simulink model "TRUAV_Dynamics_from_GTRS_trim"  (R2022b)
settings: Solver=ode4  StartTime=0.0  StopTime=3  FixedStep=0.004  RelTol=1e-3
values from neighbouring files (symbols this model uses):
  a_sound = 1116.45    [init_0_GTRS_data_Run_this_file.m]
  alpha_F_rad = alpha_F_deg * (pi/180)    [init_Vetical_2_Table.m]
  alpha_F_rad_table = alpha_F_table * (pi/180)    [init_Fuselage_Aero_Table.m]
  alpha_H_rad = alpha_H_deg * (pi/180)    [init_Horizontal_Table.m]
  alpha_HD_rad = alpha_HD_deg * (pi/180)    [init_Horizontal_C_D_Table.m]
  alpha_r0 = 0    [init_0_GTRS_data_Run_this_file.m]
  alpha_WF_epsilon_M_rad = alpha_WF_deg * pi/180    [init_WingWake_Deflection_Table.m]
  alpha_WS_CL_rad = alpha_WS_CL_deg * (pi/180)    [init_Wing_Slide_Table.m]
  b_w = 32.17    [init_0_GTRS_data_Run_this_file.m]
  beta_F_rad = beta_F_deg * (pi/180)    [init_Vetical_2_Table.m]
  beta_LD_rad_table = beta_LD_table * (pi/180)    [init_Fuselage_Aero_Table.m]
  beta_m_epsilon_M_rad = beta_m_deg * pi/180    [init_WingWake_Deflection_Table.m]
  beta_m_rad_cn = beta_m_deg_cn * pi/180    [init_Wing_Free_Table.m]
  beta_M_rad_table = beta_M_table  * (pi/180)    [init_Fuselage_Aero_Table.m]
  beta_m_S_rad = beta_m_S_deg * (pi/180)    [init_Vetical_2_Table.m]
  beta_m_WS_CL_rad = beta_m_WS_CL_deg * (pi/180)    [init_Wing_Slide_Table.m]
  beta_rad_brk = beta_KBR_rad    [init_Vetical_2_Table.m]
  beta_v_rad = beta_v_deg * (pi/180)    [init_Vetical_1_Table.m]
  beta_vD_rad = beta_vD_deg * (pi/180)    [init_Vetical_1_Table.m]
  beta_WF_Cl_rad = beta_W_deg * (pi/180)    [init_Wing_Free_Table.m]
  beta_WF_CL_rad = beta_CL_deg * (pi/180)    [init_Wing_Free_Table.m]
  beta_YlN_rad_table = beta_YlN_table * (pi/180)    [init_Fuselage_Aero_Table.m]
  c_HW = 3.92    [init_0_GTRS_data_Run_this_file.m]
  C_l_beta_CLwp_table = [ ... (first row only)    [init_Wing_Free_Table.m]
  C_l_beta_pro_CLwp_table = [ ... (first row only)    [init_Wing_Free_Table.m]
  C_L_delta_a_table = [0.00316, 0.00396, 0.00476, 0]    [init_Wing_Free_Table.m]
  C_LHB = -0.00422    [init_0_GTRS_data_Run_this_file.m]
  C_lp_C_LWP = -0.774    [init_0_GTRS_data_Run_this_file.m]
  C_m_wp_table = [ ... (first row only)    [init_Wing_Free_Table.m]
  C_MHA = 0    [init_0_GTRS_data_Run_this_file.m]
  C_MHO = 0    [init_0_GTRS_data_Run_this_file.m]
  c_R = 14/12    (= 1.16666666667)    [init_0_GTRS_data_Run_this_file.m]
  c_w = 5.225    [init_0_GTRS_data_Run_this_file.m]
  C_Y_beta = 0    [init_0_GTRS_data_Run_this_file.m]
  CD0_high_Mach_data = [0.0177, 0.0178, 0.0179, 0.0405]    [init_Wing_Free_Table.m]
  CD_4D_table = zeros(49, 4, 2, 4)    [init_Wing_Slide_Table.m]
  CDH_2D_table = zeros(length(alpha_HD_deg), length(mach_vec))    [init_Horizontal_C_D_Table.m]
  CDV_2D_table = zeros(length(beta_vD_deg), length(mach_vec))    [init_Vetical_1_Table.m]
  CL_4D_table = zeros(49, 4, 2, 4)    [init_Wing_Slide_Table.m]
  CLH_3D_table = zeros(length(alpha_H_deg), length(delta_e_deg), length(mach_vec))    [init_Horizontal_Table.m]
  CYV_3D_table = zeros(length(beta_v_deg), length(delta_r_deg), length(mach_vec))    [init_Vetical_1_Table.m]
  D_alpha_table = [D_part1, D_part2, D_part3, D_part4]    [init_Fuselage_Aero_Table.m]
  D_beta_table = [ fliplr(D_beta_half(2:end)),  D_beta_half]    [init_Fuselage_Aero_Table.m]
  D_ke = 0.24    [init_0_GTRS_data_Run_this_file.m]
  D_Kr = 0.24    [init_0_GTRS_data_Run_this_file.m]    (also in init_Vetical_1_Table.m)
  DBFO = -1.56    [init_0_GTRS_data_Run_this_file.m]
  delta_e_rad = delta_e_deg * (pi/180)    [init_Horizontal_Table.m]
  delta_r_deg = [-20, -15, 0, 15, 20]    [init_Vetical_1_Table.m]
  DLANG = -0.5    [init_0_GTRS_data_Run_this_file.m]
  epsilon_W_table = permute(epsilon_W_3D, [3, 1, 2])    [init_WingWake_Deflection_Table.m]
  flap_rad = flap_deg * (pi/180)    [init_Wing_Free_Table.m]    (also in init_Wing_Slide_Table.m)
  ft2m = 0.3048    [init_0_GTRS_data_Run_this_file.m]
  h_HW = [-0.5838, 0.01158, 0.5967, 0.002547,-2.2519]    [init_0_GTRS_data_Run_this_file.m]
  I_b = 102.5    [init_0_GTRS_data_Run_this_file.m]
  i_H = 0    [init_0_GTRS_data_Run_this_file.m]
  i_v = 0    [init_0_GTRS_data_Run_this_file.m]
  i_w = 0    [init_0_GTRS_data_Run_this_file.m]
  in2ft = 1/12    (= 0.0833333333333)    [init_0_GTRS_data_Run_this_file.m]
  Ixx = 52795    [init_0_GTRS_data_Run_this_file.m]
  Ixz = 1234    [init_0_GTRS_data_Run_this_file.m]
  Iyy = 21360    [init_0_GTRS_data_Run_this_file.m]
  Izz = 66335    [init_0_GTRS_data_Run_this_file.m]
  K1delta_data = [ ... (first row only)    [init_Wing_Free_Table.m]
  K_coeffs = [1.6 0]    [init_0_GTRS_data_Run_this_file.m]
  K_FWDF = -0.0035    [init_0_GTRS_data_Run_this_file.m]
  K_FWO = 1.4    [init_0_GTRS_data_Run_this_file.m]
  K_HNU = 0.8    [init_0_GTRS_data_Run_this_file.m]
  K_vNU = 1    [init_Vetical_1_Table.m]
  KBR_table = KBR_table_full    [init_Vetical_2_Table.m]
  Kn_delta_data = [ ... (first row only)    [init_Wing_Free_Table.m]
  Kno_delta_data = [ ... (first row only)    [init_Wing_Free_Table.m]
  L_alpha_table = [L_part1, L_part2, L_part3, L_part4]    [init_Fuselage_Aero_Table.m]
  L_beta_table = [ fliplr(L_beta_half(2:end)),  L_beta_half]    [init_Fuselage_Aero_Table.m]
  l_beta_table = [l_beta_neg, l_beta_pos]    [init_Fuselage_Aero_Table.m]
  L_n = 4.667    [init_0_GTRS_data_Run_this_file.m]
  lambda_w = -6.5*deg2rad    (= -0.11344640138)    [init_0_GTRS_data_Run_this_file.m]
  LBFO = -7.23    [init_0_GTRS_data_Run_this_file.m]
  LLANG = 0    [init_0_GTRS_data_Run_this_file.m]
  m2ft = 1/ft2m    (= 3.28083989501)    [init_0_GTRS_data_Run_this_file.m]
  M_alpha_table = [M_part1, M_part2, M_part3, M_part4]    [init_Fuselage_Aero_Table.m]
  M_beta_table = [ fliplr(M_beta_half(2:end)), M_beta_half]    [init_Fuselage_Aero_Table.m]
  Mach_brk = [0.2, 0.4, 0.5, 0.6]    [init_Wing_Free_Table.m]
  mach_vec = [0.2, 0.4, 0.5, 0.6]    [init_Horizontal_C_D_Table.m]    (also in init_Horizontal_Table.m; init_Vetical_1_Table.m)
  mass = 403.7    [init_0_GTRS_data_Run_this_file.m]
  mast_rad = mast_deg * pi/180    [init_Wing_Free_Table.m]
  MBFO = 66.5    [init_0_GTRS_data_Run_this_file.m]
  Mn_X_ke = [0 0.2 0.4 0.5 0.6 0.7]    [init_Horizontal_Table.m]
  N_beta_table = [N_beta_neg, N_beta_pos]    [init_Fuselage_Aero_Table.m]
  pos_x_CG = 300    [init_0_GTRS_data_Run_this_file.m]
  pos_x_H = 300    [init_0_GTRS_data_Run_this_file.m]
  pos_x_HW = 560    [init_0_GTRS_data_Run_this_file.m]
  pos_x_Nac = 291.7    [init_0_GTRS_data_Run_this_file.m]
  pos_x_V = 570    [init_0_GTRS_data_Run_this_file.m]
  pos_x_W = 291.7    [init_0_GTRS_data_Run_this_file.m]
  pos_y_CG = 0    [init_0_GTRS_data_Run_this_file.m]
  pos_y_H = 193    [init_0_GTRS_data_Run_this_file.m]
  pos_y_HW = 0    [init_0_GTRS_data_Run_this_file.m]
  pos_y_Nac = 193    [init_0_GTRS_data_Run_this_file.m]
  pos_y_V = 115.69    [init_0_GTRS_data_Run_this_file.m]
  pos_y_W = 96.6    [init_0_GTRS_data_Run_this_file.m]
  pos_z_CG = 81.65    [init_0_GTRS_data_Run_this_file.m]
  pos_z_H = 100    [init_0_GTRS_data_Run_this_file.m]
  pos_z_HW = 103    [init_0_GTRS_data_Run_this_file.m]
  pos_z_Nac = 118    [init_0_GTRS_data_Run_this_file.m]
  pos_z_V = 77    [init_0_GTRS_data_Run_this_file.m]
  pos_z_W = 96    [init_0_GTRS_data_Run_this_file.m]
  R = 12.5    [init_0_GTRS_data_Run_this_file.m]
  rho = 0.002376    [init_0_GTRS_data_Run_this_file.m]
  s_HW = 50.25    [init_0_GTRS_data_Run_this_file.m]
  S_max = 56    [init_0_GTRS_data_Run_this_file.m]
  S_v = 20.25    [init_0_GTRS_data_Run_this_file.m]
  S_w = 181    [init_0_GTRS_data_Run_this_file.m]
  Sidewash_4D = zeros(length(alpha_F_deg), length(beta_F_deg), length(beta_m_S_deg), length(delta_F_S_deg))    [init_Vetical_2_Table.m]
  slugft2kgm = 1.35582    [init_0_GTRS_data_Run_this_file.m]
  tau_e = 0.518    [init_0_GTRS_data_Run_this_file.m]
  tau_r = 0.27    [init_0_GTRS_data_Run_this_file.m]    (also in init_Vetical_1_Table.m)
  theta_0_R = 0.750    (= 0.75)    [init_0_GTRS_data_Run_this_file.m]
  theta_0_W = 1.187    [init_0_GTRS_data_Run_this_file.m]
  theta_twist = -41*deg2rad    (= -0.715584993318)    [init_0_GTRS_data_Run_this_file.m]
  u_max = 1181/12    (= 98.4166666667)    [init_0_GTRS_data_Run_this_file.m]
  ... (+3 more)
undefined symbols (not defined in the file or in its folder): beta_m_rad, F, Light, MIL, sigbuilder_block, tilt_cmd
libraries: simulink x2, sharedtransform x2, aerolibasang x2, aerolibwind2 x1
(part 3 of 4)

== matlab function TRUAV_Dynamics_from_GTRS_trim/Force and Moments/Propulsion1/Rotor Assembly 2 left/叶素法 ==
  data: para input; V_H input; r_n input; beta_F_params input; Psi_1 input; v_i input; a_MR input; F_b output; M_b output; delta_H input; T_NAC2B input; T_H2NAC input; ABC input; Thrust_mag output
function [F_b, M_b, Thrust_mag] = forces_moments_Left(para, V_H, r_n, beta_F_params, Psi_1, ...
                                          v_i, a_MR, delta_H, T_NAC2B, T_H2NAC,ABC)
    % ========== 左旋翼（CW）全叶素积分气动力与力矩计算 ==========
    R = para(1); theta_twist = para(2);
    rho = para(3); c = para(4); a_sound = para(5); Nb = 3;                
    
    % 同样内部取反横向周期变距，以匹配飞行控制逻辑
    theta_all = ABC(1);
    A1 = -ABC(2); B1 = ABC(3); 
    
    a0 = beta_F_params(1); a1s = beta_F_params(2); b1s = beta_F_params(3);
    delta_H = delta_H(:); % 强行拉直为 3x1 列向量
    
    N_segments = 40;
    dr = R / N_segments;
    r_vec = (0.5:1:N_segments-0.5)' * dr; 
    x = r_vec / R;
    
   % 初始化整个旋翼在桨毂系(Hub)下的总力和总力矩
    F_HUB_total = zeros(3,1); 
    M_HUB_total = zeros(3,1); 
    
    % ========== 改造点：方位角离散平均法 ==========
    N_azimuth = 36; % 将一圈分为 36 份 (每 10 度算一次)
    dPsi = 2 * pi / N_azimuth;
    
    for k = 1:N_azimuth
        % 虚拟桨叶当前的方位角
        Psi = (k - 1) * dPsi; 
        
        % 根据傅里叶级数实时计算该方位角下的挥舞角和角速度
        beta = a0 - a1s*cos(Psi) - b1s*sin(Psi);
        beta_dot = r_n * (a1s*sin(Psi) - b1s*cos(Psi));
        
        dY_prime = zeros(N_segments, 1);
        dZ_prime = zeros(N_segments, 1);
        dQ_torque = zeros(N_segments, 1); 
        
        % ========== 2. 逐段计算叶素气动力 ==========
        for i = 1:N_segments
            r_local = r_vec(i);
            
            % 【左旋翼 CW 的正确面内速度分解】
            % 注意这里和右旋翼的区别！
            U_T = r_n * r_local + V_H(1) * sin(Psi) - V_H(2) * cos(Psi); 
            U_R = V_H(1) * cos(Psi) + V_H(2) * sin(Psi);
            
            U_P = r_local * beta_dot + U_R * beta + V_H(3) + v_i;
            
            if U_T < 0; U_T = abs(U_T); end
            
            phi_b = atan2(U_P, U_T);
            % 注意：左旋翼在函数开头应该已经把 A1 内部取反了 (A1 = -ABC(2))
            theta = theta_all + A1*cos(Psi) + B1*sin(Psi) + theta_twist*x(i);
            alpha_blade = theta - phi_b;
            
            U = sqrt(U_T^2 + U_P^2);
            M_local = U / a_sound;
            abs_alpha = abs(alpha_blade);
            
            % 阻力系数经验公式
            cd_base = 0.015 + abs_alpha * (0.068 + abs_alpha * 0.81);
            comp_term = 0.01 * abs_alpha + 0.02 *(0.85+ max(M_local,0.35)); 
            cd_comp = max(0, comp_term);
            cd_local = min(0.11, cd_base + cd_comp);
            
            dL = 0.5 * rho * U^2 * a_MR * alpha_blade * c * dr;
            dD = 0.5 * rho * U^2 * cd_local * c * dr;
            
            % 桨叶主轴系气动力
            dY_prime(i) = dL * sin(phi_b) + dD * cos(phi_b);
            dZ_prime(i) = dL * cos(phi_b) - dD * sin(phi_b);
            dQ_torque(i) = dY_prime(i) * r_local; 
        end
        
        Y_prime = sum(dY_prime);   
        Z_prime = sum(dZ_prime);   
        Q_blade = sum(dQ_torque);  
        
        % 顺时针旋转的局部受力向量 (阻力始终与切向速度相反)
        F_blade_local = [0; -Y_prime; Z_prime]; 
        
        % ========== 3. 坐标转换：桨叶系 -> 挥舞系 -> 桨毂系 ==========
        
        % 3.1 【已修复】挥舞矩阵 (绕 Y 轴向上翘起 beta)
        T_Flap2Rot = [ cos(beta),  0, -sin(beta);
                               0,  1,          0;
                       sin(beta),  0,  cos(beta)];
        
        % 3.2 顺时针(CW)旋转的特征坐标转换矩阵
        T_Rot2Hub = [ cos(Psi), sin(Psi), 0;
                     -sin(Psi), cos(Psi), 0;
                             0,        0, 1];
                        
        % 单根桨叶力转换到桨毂固定系
        F_HUB_blade = T_Rot2Hub * T_Flap2Rot * F_blade_local;
        
        % 累加这个方位角切片上的力
        F_HUB_total = F_HUB_total + F_HUB_blade;

        Thrust_mag = abs(F_HUB_total(3));
        
        % 累加反扭矩：左旋翼(CW)的气动反扭矩阻碍旋转，方向为 +Z
        M_HUB_total(3) = M_HUB_total(3) - Q_blade; 
    end
    
    % ========== 4. 求一圈的平均力，再乘以真实桨叶数 ==========
    % 因为我们积了 36 次，相当于有 36 片桨叶，所以要除以 36，再乘以真实的 3 片
    F_HUB_total = F_HUB_total * (Nb / N_azimuth);
    M_HUB_total = M_HUB_total * (Nb / N_azimuth);
    
    % ========== 5. 转换到机体轴系 (Body Frame) ==========
    T_HUB2BODY = T_NAC2B * T_H2NAC; 
    F_b = T_HUB2BODY * F_HUB_total;
    M_hub_body = T_HUB2BODY * M_HUB_total;
    
    % ========== 6. 计算最终重心的总力矩 ==========
    M_b = M_hub_body + cross(delta_H, F_b);
  end

== matlab function TRUAV_Dynamics_from_GTRS_trim/6DOF Model/disturbance2/noise Disturb1 ==
  data: n input; t input; y output
function y = fcn(n, t)
    if t>=7&&t<=14
        y=n;
    else
        y=0*n;
    end
end

== matlab function TRUAV_Dynamics_from_GTRS_trim/6DOF Model/disturbance2/noise Disturb2 ==
  data: n input; t input; y output
function y = fcn(n, t)
    if t>=19&&t<=23
        y=n;
    else
        y=0*n;
    end
end

== matlab function TRUAV_Dynamics_from_GTRS_trim/Force and Moments/Propulsion1/Rotor Assembly 2 left/旋转矩阵计算 ==
  data: T_H2NAC output; tilt input; T_NAC2B output
function [T_H2NAC ,T_NAC2B]  = Transf(tilt)

T_H2NAC = [-1     0     0;
          0     1     0;
          0     0     -1];

T_NAC2B = [cos(tilt)  0     -sin(tilt);
           0          1       0;
           sin(tilt)  0     cos(tilt)];

== matlab function TRUAV_Dynamics_from_GTRS_trim/6DOF Model/MATLAB Function ==
  data: Ib input; F input; M input; V_b input; wbe_b input; Eu input; d1 input; x1to3dot output; x4to6dot output; x7to9dot output; d2 input
function [x1to3dot,x4to6dot,x7to9dot] = EuFcn(Ib,F,M,V_b,wbe_b,Eu,d1,d2)

p=wbe_b(1);q=wbe_b(2);r=wbe_b(3);
Ix=Ib(1);Iy=Ib(2);Iz=Ib(3);Ixz=Ib(4);
Ibb=[Ix 0 Ixz;
    0 Iy 0;
    Ixz 0 Iz];
Mx = M(1);My = M(2);Mz = M(3);

x7=Eu(1);
x8=Eu(2);
%-----------------10. STATE DERIVATIVES--------------------------    
 %Form F_b (all the forces in Fb) and calculate udot, vdot, wdot
 x1to3dot=(1/403.7)*F-cross(wbe_b,V_b)+(1/403.7)*d1;
 
 %Form Mcg_b (all moment about CoG in Fb) and calculate pdot, qdot, rdot.
%  invIb=inv(Ib);
 x4to6dot=Ibb\(M-cross(wbe_b,Ibb*wbe_b)+d2);
 
 %Calculate phidot, thetadot, and psidot
 R_omega=[1 sin(x7)*tan(x8) cos(x7)*tan(x8);
        0 cos(x7) -sin(x7);
        0 sin(x7)/cos(x8) cos(x7) /cos(x8)];
%  H_phi=[0 cos(x7) -sin(x7);
%         0 sin(x7)/cos(x8) cos(x7) /cos(x8);
%         1 sin(x7)*tan(x8) cos(x7)*tan(x8)];  
 x7to9dot=R_omega*wbe_b;

== matlab function TRUAV_Dynamics_from_GTRS_trim/6DOF Model/MATLAB Function3 ==
  data: R_be output; Par_b input; Par_e output; Eu input
function [R_be,Par_e]= EuFcn(Par_b,Eu)

phi=Eu(1);theta=Eu(2);psi=Eu(3);



R_be = [cos(theta)*cos(psi), sin(phi)*sin(theta)*cos(psi)-cos(phi)*sin(psi), sin(phi)*sin(psi)+cos(phi)*sin(theta)*cos(psi);
        cos(theta)*sin(psi), sin(phi)*sin(theta)*sin(psi)+cos(phi)*cos(psi), -sin(phi)*cos(psi)+cos(phi)*sin(theta)*sin(psi);
        -sin(theta), sin(phi)*cos(theta), cos(phi)*cos(theta)];

Par_e=R_be*Par_b;
 
for i=1:1:9
      if isnan(R_be(i))
         Par_e(i)= double(isnan(Par_e(i)));
      end
end

== matlab function TRUAV_Dynamics_from_GTRS_trim/6DOF Model/disturbance1/Disturb4 ==
  data: t input; y output
function y = fcn(t)
    y=1+2*sin(1.5*pi*t)+cos(0.5*pi*t);
    
end

== matlab function TRUAV_Dynamics_from_GTRS_trim/6DOF Model/disturbance1/Disturb1 ==
  data: t input; y output
function y = fcn(t)
    y=2+1.5*cos(2*pi*t)+sin(0.3*pi*t);
%     if t>=8&&t<=14
%         y=y1*(1+sin(1/6*pi*(t-8)));
%     elseif t>=21&&t<=23
%         y=y1*(1+sin(1/2*pi*(t-21)));
%     else 
%         y=y1;
%     end
end

== matlab function TRUAV_Dynamics_from_GTRS_trim/6DOF Model/disturbance1/Disturb2 ==
  data: t input; y output
function y = fcn(t)
    y=-2+1.5*sin(pi*t)+2*cos(3*pi*t);
%     if t>=8&&t<=14
%         y=y1*(1+sin(1/6*pi*(t-8)));
%     elseif t>=21&&t<=23
%         y=y1*(1+sin(1/2*pi*(t-21)));
%     else 
%         y=y1;
%     end
end

== matlab function TRUAV_Dynamics_from_GTRS_trim/6DOF Model/disturbance1/noise Disturb1 ==
  data: n input; t input; y output
function y = fcn(n, t)
    if t>=7&&t<=14
        y=n;
    else
        y=0*n;
    end
end

== matlab function TRUAV_Dynamics_from_GTRS_trim/6DOF Model/disturbance1/noise Disturb2 ==
  data: n input; t input; y output
function y = fcn(n, t)
    if t>=19&&t<=23
        y=n;
    else
        y=0*n;
    end
end

== matlab function TRUAV_Dynamics_from_GTRS_trim/6DOF Model/限制在±180度 ==
  data: x input; y output
function y = fcn(x)
x = mod(x,2*pi);
y = x.*(0<=x & x <= pi) + (x - 2*pi).*(pi<x & x<2*2*pi);  % x in (-pi,pi]

== matlab function TRUAV_Dynamics_from_GTRS_trim/Force and Moments/body/Fuselage/机身气动力 ==
  data: q_F output; para input; V_body input; alpha_rad output; beta_rad output
function [q_F, alpha_rad, beta_rad] = f_kinematics(para, V_body)
    % =====================================================================
    % 机身拆分模块 1：运动学解算 (算出迎角、侧滑角与动压)
    % ---------------------------------------------------------------------
    % 【输出说明】
    % alpha_rad : 机身迎角 (rad)，输出给外部 Alpha 查表模块
    % beta_rad  : 机身侧滑角 (rad)，输出给外部 Beta 查表模块
    % q_F       : 机身动压 (lb/ft^2)，直接传递给第二个模块
    % =====================================================================
    
    rho = para(1);  
         
    % 计算局部相对速度
    V_local = V_body;
    u = V_local(1); 
    v = V_local(2); 
    w = V_local(3);
    
    V_mag = norm(V_local); 
    
    % 求解角度与动压
    if V_mag < 0.1
        alpha_rad = 0;
        beta_rad  = 0;
        q_F       = 0;
    else
        alpha_rad = atan2(w, u);
        v_ratio = max(min(v / V_mag, 1), -1); 
        beta_rad  = asin(v_ratio);
        q_F = 0.5 * rho * V_mag^2;
    end
end

== matlab function TRUAV_Dynamics_from_GTRS_trim/Force and Moments/body/Fuselage/机身气动力1 ==
  data: para input; q_F input; F_b output; M_b output; alpha_rad input; beta_rad input; aero_alpha input; aero_beta input
function [F_b, M_b] = F_M_f(para, q_F, alpha_rad, beta_rad, aero_alpha, aero_beta)
    % =====================================================================
    % 机身拆分模块 2：动力学合成 (接收查表结果，算出总力和力矩)
    % ---------------------------------------------------------------------
    % 
    % aero_alpha : [3x1] 外部 Alpha 查表结果打包 [L_alpha_0; D_alpha_0; M_alpha_0]
    % aero_beta  : [3x1] 外部 Beta 查表结果打包 [L_beta; D_beta; M_beta]
    % =====================================================================
    
    LBFO  = para(2); 
    LLANG = para(3); 
    DBFO  = para(4); 
    DLANG = para(5); 
    MBFO  = para(6); 
    
    
    
    % 1. 解析外部查表传入的数据
    L_alpha_0 = aero_alpha(1); 
    D_alpha_0 = aero_alpha(2); 
    M_alpha_0 = aero_alpha(3); 
    
    L_beta = aero_beta(1); 
    D_beta = aero_beta(2); 
    M_beta = aero_beta(3); 
    Y_beta = aero_beta(4); 
    l_beta = aero_beta(5); 
    N_beta = aero_beta(6); 
         
    % 2. 核心经验公式计算
    cos2_beta = (cos(beta_rad))^2;
    
    L_F       = q_F * ( L_alpha_0 * cos2_beta + L_beta + LBFO + LLANG );
    D_F       = q_F * ( D_alpha_0 * cos2_beta + D_beta + DBFO + DLANG );
    Y_F_prime = q_F * Y_beta;
    
    M_F_prime = q_F * ( M_alpha_0 * cos2_beta + M_beta + MBFO );
    l_F_prime = q_F * l_beta;
    N_F_prime = q_F * N_beta;
    
    % 3. 风轴向机体轴 3D 转换
    sa = sin(alpha_rad); ca = cos(alpha_rad);
    sb = sin(beta_rad);  cb = cos(beta_rad);
    
    F_body = zeros(3,1);
    F_body(1) = -D_F * ca * cb - Y_F_prime * ca * sb + L_F * sa;
    F_body(2) = -D_F * sb      + Y_F_prime * cb;
    F_body(3) = -D_F * sa * cb - Y_F_prime * sa * sb - L_F * ca;
    
    M_profile = zeros(3,1);
    M_profile(1) =  l_F_prime * ca - N_F_prime * sa;
    M_profile(2) =  M_F_prime; 
    M_profile(3) =  l_F_prime * sa + N_F_prime * ca;
    
    % 4. 平行轴定理向重心搬移
    M_b = M_profile;
    F_b = F_body;
end

== matlab function TRUAV_Dynamics_from_GTRS_trim/Force and Moments/Propulsion1/Rotor Assembly 2 left/计算挥舞角、桨尖马赫数 桨叶升力线斜率1 ==
  data: para input; V input; beta_F_Para output; r_n input; tilt input; mu input; AB input; alpha input; pqr input; v_1d input; M_tip output; a_MR output; lamda input
function [beta_F_Para, M_tip, a_MR] = rotor_cal1(...
    para, V, r_n, tilt, mu, AB, alpha, pqr, v_1d, lamda)
% 整合旋翼气动与挥舞计算模型（包含洛克数自动计算）
% 输入：
%   para     - 参数向量 [R, theta_0_W, theta_0_R, theta_twist, a_sound, alpha_0, rho, c, I_b]
%              R: 旋翼半径 [ft]
%              theta_0_W: 悬停总距 [rad]（对应β_M=0）
%              theta_0_R: 悬停总距 [rad]（对应β_M=90°）
%              theta_twist: 桨叶线性扭转率 [rad]
%              a_sound: 当地声速 [ft/s]
%              alpha_0: 桨叶零升迎角修正 [rad]
%              rho: 空气密度 [slug/ft³]
%              c: 桨叶弦长 [in]（自动转换为ft）
%              I_b: 桨叶挥舞惯性矩 [slug·ft²]
%   V        - 飞机前进速度 [ft/s]
%   r_n      - 展向位置比率（通常为1，代表桨尖）
%   tilt   - 短舱倾角 [rad]
%   mu       - 前进比（无量纲）
%   AB       - 周期变距向量 [A1, B1]  [rad]
%   alpha    - 迎角[rad]
%   gamma_b  - 洛克数（占位符，实际会被覆盖计算，可任意值）
%   pqr      - 机体角速度 [p,q,r] [rad/s]
%   lamda    - 入流比（未使用，保留接口）
%   Psi    - 方位角 [rad]
% 输出：
%   beta_F     - 挥舞角 [rad]
%   M_tip    - 桨尖马赫数
%   a_MR     - 旋翼升力线斜率 [1/rad]

% 解析参数
R = para(1);
theta_0_W = para(2);
theta_0_R = para(3);
theta_twist = para(4);
a_sound = para(5);
alpha_0 = para(6);
rho = para(7);
c = para(8);
I_b = para(9);

p = pqr(1);
q = pqr(2);
A1 = AB(2);
B1 = AB(3);

% ========== 1. 计算桨尖马赫数 M_tip ==========
V_tip = sqrt(V^2 + (r_n*R)^2 + 2*V*r_n*R*cos(tilt));
M_tip = V_tip / a_sound;

% ========== 2. 计算升力线斜率 a_MR（Kleinhesselink 论文）==========
denom = sqrt(1 - (0.75*M_tip)^2 * sin(tilt));
if denom < 1e-6
    denom = 1e-6;
end
 a_MR = (4.95 + mu * (8 + 30*mu)) / denom;

% ========== 3. 计算洛克数 gamma ==========
gamma_b_calc = rho * a_MR * c * R^4 / I_b;   % 无量纲洛克数

% ========== 4. 计算挥舞角 ==========
theta0 = 2*(tilt)/pi * (theta_0_W - theta_0_R) + theta_0_R;
alpha_s = alpha - tilt;

% ... (前面的 M_tip 和 洛克数 计算保持不变) ...

% 4.1 后倒角 a1s（纵向挥舞）- 陀螺耦合项 p, q 符号取反
term1 = (2*mu) / (1 - 0.5*mu^2);
term2 = (4/3)*theta0 + theta_twist + mu*alpha_s - v_1d/(r_n*R);
term3 = - (1 + 1.5*mu^2) / (1 - 0.5*mu^2) * B1;
% 【修正】：q 变正，p 变负
term4 = 16/gamma_b_calc * q / r_n - p / r_n; 
a1s = term1 * term2 + term3 + term4/(1 - 0.5*mu^2);

% 4.2 侧倒角 b1s（横向挥舞）- 陀螺耦合项 p, q 符号取反
term1_b = (2*mu) / (1 + 0.5*mu^2);
term2_b = (4/3) * mu * alpha_0;
term3_b = A1; 
% 【修正】：p 变正，q 变正
term4_b = 16/gamma_b_calc * p / r_n;
term5_b = q / r_n;
b1s = term1_b * term2_b + term3_b + (term4_b + term5_b)/(1 + 0.5*mu^2);

% 锥度角 a0（简化）
gamma_used = gamma_b_calc;   % 使用计算得到的洛克数
a0 = (gamma_used/8) * ((4/3)*theta0*(1 + mu^2) + 2*lamda*mu);

% 挥舞角随方位角变化
beta_F_Para = [a0 a1s b1s];

end

== matlab function TRUAV_Dynamics_from_GTRS_trim/Force and Moments/body/Horizontal/平尾气动力1 ==
  data: para input; CG input; AC_t input; tilt input; Ke_coeffs input; q_H input; alpha_body_t input; F_b output; M_b output; beta_t input; alpha_HL input; C_LH input; C_DH input
function [F_b, M_b] = tail_dynamics(para, CG, AC_t, tilt, Ke_coeffs, q_H, alpha_body_t, beta_t, alpha_HL, C_LH, C_DH)
    
    % =====================================================================
    % 平尾拆分模块 2：动力学合成
    % ---------------------------------------------------------------------
    % 【输入说明】
    % alpha_HL   : 需要用来计算俯仰力矩 Pitch_stab
    % C_LH, C_DH : 外部 3-D Lookup Table 查得的升力/阻力系数
    % =====================================================================
    
    S_H = para(2); c_H = para(3);
    
    % NASA 绝对坐标转换为 NED 相对力臂 (X前, Y右, Z下)
    r_ac_x = CG(1) - AC_t(1); 
    r_ac_y = AC_t(2) - CG(2); 
    r_ac_z = CG(3) - AC_t(3); 
    
    r_ac = [r_ac_x; r_ac_y; r_ac_z];
    
    % 【修复Bug】: 提取修正后的力矩系数索引
    C_LHB = Ke_coeffs(3); 
    C_MHO = Ke_coeffs(5); % 原为4，现修正为5
    C_MHA = Ke_coeffs(6); % 原为5，现修正为6
    
    % 1. 计算总升力系数
    beta_limit = min(15, abs(beta_t * 180/pi)); 
    C_L_wdot = 0; w_dot = 0; % 预留非定常接口
    
    C_LH_total = C_LH + C_L_wdot * w_dot + C_LHB * beta_limit * cos(tilt);
    
    % 2. 气动力计算
    Lift = q_H * S_H * C_LH_total;
    Drag = q_H * S_H * C_DH;
    Side = 0; 
    
    % 3. 风轴向机体轴 3D 转换
    sa = sin(alpha_body_t); ca = cos(alpha_body_t);
    sb = sin(beta_t);       cb = cos(beta_t);
    
    F_body = [-Drag*ca*cb - Side*ca*sb + Lift*sa;
              -Drag*sb      + Side*cb;
              -Drag*sa*cb - Side*sa*sb - Lift*ca];
          
    % 4. 俯仰力矩计算与搬移
    Pitch_stab = q_H * S_H * c_H * (C_MHO + C_MHA * alpha_HL);
    M_profile = [0; Pitch_stab; 0];
    
    M_b = M_profile + cross(r_ac, F_body);
    F_b = F_body;
end

== matlab function TRUAV_Dynamics_from_GTRS_trim/Force and Moments/body/Horizontal/平尾气动力2 ==
  data: para input; V_mag_t input; epsilon_w input; delta_e input; V_local_t input; alpha_HL output; alpha_HD output; Ke_coeffs input; X_Ke input; q_H output; alpha_body_t output; beta_t output; Mach_N input
function [alpha_HL, alpha_HD, q_H, alpha_body_t, beta_t] = tail_kinematics(para,  V_mag_t, epsilon_w, delta_e,  V_local_t , Ke_coeffs, X_Ke, Mach_N)
    
    % =====================================================================
    % 平尾拆分模块 1：运动学与气动迎角解算
    % ---------------------------------------------------------------------
    % 【注意】：X_Ke 必须在外部通过马赫数先行查表后，作为输入传入本模块！
    % 
    % 【输出说明】
    % alpha_HL, alpha_HD, Mach_N : 输出给外部 3-D Lookup Table 查 C_LH 和 C_DH
    % V_wake_tail_RL             : 输出给【垂尾】的运动学模块
    % q_H, alpha_body_t, beta_t  : 传递给平尾模块 2 (tail_dynamics)
    % =====================================================================
    
    rho = para(1); i_H = para(4); 
             
                      
        
    % 2. 局部速度计算
    
    
    u_t = V_local_t(1); v_t = V_local_t(2); w_t = V_local_t(3);
   
    
    % 【修复Bug】: 重新定义索引 4 为 K_HNU
    K_HNU = Ke_coeffs(4); 
    
    if V_mag_t < 0.1
        alpha_body_t = 0; beta_t = 0; q_H = 0;
    else
        alpha_body_t = atan2(w_t, u_t);
        beta_t = asin(max(min(v_t / V_mag_t, 1), -1));
        q_H = 0.5 * K_HNU * rho * V_mag_t^2;
    end
    
    % 3. 升降舵非线性舵效计算
    D_Ke = Ke_coeffs(1); tau_e = Ke_coeffs(2);
    delta_e_deg = delta_e * (180/pi); 
    
    if abs(delta_e_deg) <= 15
        K_e = X_Ke; % 使用外部传入的查表结果
    else
        K_e = X_Ke - D_Ke * ((abs(delta_e_deg) - 15) / 15);
    end
    elevator_effect = K_e * tau_e * delta_e;
    
    % 4. 气动迎角计算 (马赫数死区)
    if Mach_N < 0.2
        alpha_HL = alpha_body_t + i_H - epsilon_w;
    else
        alpha_HL = alpha_body_t + i_H - epsilon_w + elevator_effect;
    end
    
    alpha_HD = alpha_body_t + i_H - epsilon_w + elevator_effect; 
end

== matlab function TRUAV_Dynamics_from_GTRS_trim/Force and Moments/body/Horizontal/平尾气动力3 ==
  data: para input; V_body input; pqr input; CG input; Mach_H output; AC_t input; v_i_RL input; tilt input; h_coeffs input; V_wake_tail_RL output; V_mag_t output; V_local_t output
function [Mach_H, V_wake_tail_RL, V_mag_t, V_local_t] = tail_Mach(para, V_body, pqr, CG, AC_t, v_i_RL, tilt, h_coeffs)
    
    % =====================================================================
    % 平尾拆分模块 1：运动学与气动迎角解算
    % ---------------------------------------------------------------------
    % 【注意】：X_Ke 必须在外部通过马赫数先行查表后，作为输入传入本模块！
    % 
    % 【输出说明】
    % alpha_HL, alpha_HD, Mach_N : 输出给外部 3-D Lookup Table 查 C_LH 和 C_DH
    % V_wake_tail_RL             : 输出给【垂尾】的运动学模块
    % q_H, alpha_body_t, beta_t  : 传递给平尾模块 2 (tail_dynamics)
    % =====================================================================
       
    a_sound = para(5); 
             
    % 1. 旋翼诱导速度衰减
    u = V_body(1); 
    beta_M_deg = tilt * (180/pi); 
    
    h0 = h_coeffs(1); h1 = h_coeffs(2); h2 = h_coeffs(3); 
    h3 = h_coeffs(4); h4 = h_coeffs(5);
    
    vel_ratio = (u - 168.89 + h4 * beta_M_deg) / 168.89;
    K_h = (h0 + h1 * beta_M_deg + (h2 + h3 * beta_M_deg) * vel_ratio^2);
    v_i_tail_RL = K_h * v_i_RL; 
    
    % 输出给-----垂尾------使用的尾流矩阵
    V_wake_tail_RL = [v_i_tail_RL(1)*sin(tilt), v_i_tail_RL(2)*sin(tilt);
                      0,                        0;
                      -v_i_tail_RL(1)*cos(tilt), -v_i_tail_RL(2)*cos(tilt)];
                  
    V_wake_tail_avg = mean(V_wake_tail_RL, 2);
    
    % 2. 局部速度计算
    
    % 【修复】：NASA 绝对坐标转换为 NED 相对力臂 (X前, Y右, Z下)
    r_ac_x = CG(1) - AC_t(1); % FS重心 - FS气动中心
    r_ac_y = AC_t(2) - CG(2); % BL气动中心 - BL重心
    r_ac_z = CG(3) - AC_t(3); % WL重心 - WL气动中心
    
    r_ac = [r_ac_x; r_ac_y; r_ac_z];
    
    V_local_t = V_body + cross(pqr, r_ac) + V_wake_tail_avg;
        
    V_mag_t = norm(V_local_t);

    Mach_H = V_mag_t / a_sound;
    
    
end

== matlab function TRUAV_Dynamics_from_GTRS_trim/Force and Moments/body/Vertical/垂尾气动力 ==
  data: para input; V_body input; Mach_N output
function Mach_N = vtail_prep(para, V_body)
    % =====================================================================
    % 垂尾拆分模块 1：状态预处理 (算出马赫数，用于驱动第一级 X_Kr 查表)
    % =====================================================================
    a_sound = para(4); % 提取音速
    Mach_N = norm(V_body) / a_sound;
end

== matlab function TRUAV_Dynamics_from_GTRS_trim/Force and Moments/body/Vertical/垂尾气动力1 ==
  data: para input; CG input; AC_v_R input; delta_r input; Kr_coeffs input; q_v input; alpha_xz input; F_b output; M_b output; beta_local input; K_r input; Mach_N input; CY_v_0 input; CY_v_delta input; CD_v input; K_beta_R_in input; Sidewash_factor input
function [F_b, M_b] = vtail_dynamics(para, CG, AC_v_R, delta_r, Kr_coeffs, ...
          q_v, alpha_xz, beta_local, K_r, Mach_N, ...
          CY_v_0, CY_v_delta, CD_v, K_beta_R_in, Sidewash_factor)
      
    % =====================================================================
    % 垂尾拆分模块 3：动力学合成 (内部自动处理双尾翼对称计算)
    % ---------------------------------------------------------------------
    % 【输入要求】
    % AC_v_R   : [3x1] 仅需输入右侧垂尾气动中心
    % K_beta_R_in : 支持 [1x1] 标量 或 [2x1] 向量
    % =====================================================================
    
    S_v = para(2); 
    % 内部自动镜像生成左侧垂尾气动中心，并打包为 3x2 矩阵
    AC_v_L = [AC_v_R(1); -AC_v_R(2); AC_v_R(3)];
    AC_v_list = [AC_v_R, AC_v_L]; 
    
    num_fins = 2; 
    tau_r = Kr_coeffs(2);
    a_v = 4.0; % M_N > 0.2 时的经验导数斜率
    
    Total_Force = zeros(3,1);
    Total_Moment = zeros(3,1);
    
    for i = 1:num_fins
        r_ac_x = CG(1) - AC_v_list(1, i); 
        r_ac_y = AC_v_list(2, i) - CG(2); 
        r_ac_z = CG(3) - AC_v_list(3, i); 
        
        r_ac = [r_ac_x; r_ac_y; r_ac_z];
        
        % 解析对应侧的查表系数
        CY0 = CY_v_0(i);
        CY_dr = CY_v_delta(i);
        CD = CD_v(i);
        
        % 维度自适应：如果传进来的是标量就共用，是向量就分别读取
        if length(K_beta_R_in) == 1
            K_beta_R = K_beta_R_in;
        else
            K_beta_R = K_beta_R_in(i);
        end
        
        % 气动系数衰减与马赫分段逻辑
        if Mach_N <= 0.2 
            C_Yv = CY0 * (K_beta_R * Sidewash_factor) + (CY_dr - CY0);
        else
            C_Yv = CY0 * (K_beta_R * Sidewash_factor) + a_v * K_r * tau_r * delta_r;
        end
        
        % 阻力系数侧洗衰减 
        C_Dv_total = CD * (K_beta_R * Sidewash_factor);
        
        % 局部风轴系气动力
        Side_wind = -C_Yv * q_v(i) * S_v; 
        Drag_wind = C_Dv_total * q_v(i) * S_v;
        
        % 风轴向机体轴 3D 转换
        sa = sin(alpha_xz(i)); ca = cos(alpha_xz(i));
        sb = sin(beta_local(i)); cb = cos(beta_local(i));
        
        F_body_v = [-Drag_wind*ca*cb - Side_wind*ca*sb;
                    -Drag_wind*sb    + Side_wind*cb;
                    -Drag_wind*sa*cb - Side_wind*sa*sb];
                
        Total_Force = Total_Force + F_body_v;
        % 叉乘产生绕重心的力矩！
        Total_Moment = Total_Moment + cross(r_ac, F_body_v);
    end
    
    F_b = Total_Force;
    M_b = Total_Moment;
end

== matlab function TRUAV_Dynamics_from_GTRS_trim/Force and Moments/body/Vertical/垂尾气动力2 ==
  data: para input; V_body input; pqr input; CG input; beta_v output; beta_vD output; AC_v_R input; V_wake_tail_RL input; delta_r input; Kr_coeffs input; X_Kr input; q_v output; K_r output; alpha_xz output; beta_local output; V_T output
function [beta_v, beta_vD, q_v, K_r, alpha_xz, beta_local, V_T] = vtail_kinematics(para, V_body, pqr, CG, AC_v_R, V_wake_tail_RL, delta_r, Kr_coeffs, X_Kr)
    
    % =====================================================================
    % 垂尾拆分模块 2：运动学与气动角度解算 (内部自动处理双垂尾对称)
    % ---------------------------------------------------------------------
    % 【输入修改说明】
    % AC_v_R   : [3x1] 仅需输入右侧垂尾的气动中心坐标
    % =====================================================================
    
    rho = para(1); i_v = para(3);
    
    % 【核心修改】：内部自动利用镜像对称生成左垂尾，并拼装为 3x2 矩阵
    % 假设标准坐标系下，右侧 y 为正，左侧 y 为负
    AC_v_L = [AC_v_R(1); -AC_v_R(2); AC_v_R(3)];
    AC_v_list = [AC_v_R, AC_v_L]; % 第1列为右垂尾(i=1)，第2列为左垂尾(i=2)
    num_fins = 2; % 固定为双垂尾
    
    % 提取机身全局参数 (用于供外部查侧洗系数)
    u_cg = V_body(1);
    V_T = norm(V_body);
        
    % 参数提取 (注意将 K_vNU 加入数组)
    D_Kr = Kr_coeffs(1); tau_r = Kr_coeffs(2); K_vNU = Kr_coeffs(3); 
    
    % 方向舵非线性舵效 K_r
    delta_r_deg = delta_r * (180/pi);
    if abs(delta_r_deg) <= 15 
        K_r = X_Kr; % 使用第一级查表值
    else
        K_r = X_Kr - D_Kr * ((abs(delta_r_deg) - 15) / 15); 
    end
    
    % 初始化 [2x1] 列向量 (1对应右，2对应左)
    beta_v = zeros(2,1); beta_vD = zeros(2,1); q_v = zeros(2,1);
    alpha_xz = zeros(2,1); beta_local = zeros(2,1);
    
    for i = 1:num_fins
        % NASA 绝对坐标转换为 NED 相对力臂 (X前, Y右, Z下)
        r_ac_x = CG(1) - AC_v_list(1, i); % FS重心 - FS气动中心 (垂尾在后，算出负值)
        r_ac_y = AC_v_list(2, i) - CG(2); % BL气动中心 - BL重心 
        r_ac_z = CG(3) - AC_v_list(3, i); % WL重心 - WL气动中心 (垂尾在上，算出负值)
        
        r_ac = [r_ac_x; r_ac_y; r_ac_z];
        % 提取对应侧的尾迹流场 (必须保证 V_wake_tail_RL 也是第一列右、第二列左)
        V_local_v = V_body + cross(pqr, r_ac) + V_wake_tail_RL(:, i);
        
        U_v = V_local_v(1); V_v = V_local_v(2); W_v = V_local_v(3);
        V_mag_v = norm(V_local_v); 
        
        % U_v 速度下限死区保护 (PDF Eq. D)
        if abs(U_v) < 35
            U_v_eff = 35 * sign(U_v);
            if U_v_eff == 0; U_v_eff = 35; end 
        else
            U_v_eff = U_v;
        end
        
        % 纯几何侧滑角 
        beta_v(i) = -i_v + atan2(V_v, sqrt(U_v_eff^2 + W_v^2));
        
        % 阻力计算用侧滑角 
        beta_vD(i) = beta_v(i) + K_r * tau_r * delta_r;
        
        % 动压计算
        if u_cg >= 0 && abs(V_v/V_mag_v) < 1
            eta_vs = 0.95; 
        else
            eta_vs = 1.0;  
        end
        q_v(i) = 0.5 * rho * K_vNU * eta_vs * V_mag_v^2;
        
        % 投影角度计算
        if V_mag_v < 0.1
            alpha_xz(i) = 0; beta_local(i) = 0;
        else
            alpha_xz(i) = atan2(W_v, U_v);
            beta_local(i) = asin(max(min(V_v / V_mag_v, 1), -1));
        end
    end
end

== matlab function TRUAV_Dynamics_from_GTRS_trim/Force and Moments/Propulsion1/Rotor Assembly 2 left/桨毂中心速度、前进比、 侧滑角、入流比、诱导速度 ==
  data: Para input; V_H output; tilt input; CG input; CT input; mu output; beta_w output; omega input; r_n input; V_body input; T_H2NAC input; lamda output; v_i output; POS_H output; T_NAC2B input
function [V_H, mu, beta_w, lamda, v_i, POS_H] = fcn(Para, tilt, CG, CT, omega, r_n, V_body, T_H2NAC, T_NAC2B)

    % ========== 解析结构参数 ==========
    SL_SP = Para(1);     % 枢轴点纵向位置 [in]
    BL_SP = Para(2);     % 枢轴点横向位置 [in]
    WL_SP = Para(3);     % 枢轴点垂向位置 [in]
    L_n = Para(4);  
    R = Para(5);
    
    Omega_R = r_n * R;   % 预计算桨尖速度

   % ========== 计算桨毂中心绝对位置 (NASA 体系) ==========
    % x_H 公式没问题：倾转 90 度时，桨毂向前伸出 L_n，FS 变小
    x_H = SL_SP - L_n * sin(tilt); 
    
    y_H = BL_SP; 
    
    % z_H 必须修正：直升机模式 (tilt=0) 时最高，固定翼模式 (tilt=90) 时放平
    z_H = WL_SP + L_n * cos(tilt);

    % ========== 计算重心与桨毂中心相对位置 ==========
    x_BH = CG(1) - x_H;
    y_BH = -CG(2) + y_H;                  % [in]
    z_BH = CG(3) - z_H;                  % [in]

    POS_H = [x_BH;y_BH;z_BH];

    % ========== 计算桨毂中心速度（桨毂系） ==========
%     Omega_skew = [ 0,         omega(3),  -omega(2);
%                   -omega(3),  0,          omega(1);
%                    omega(2), -omega(1),   0 ];
               
    % 先求出机体坐标系下的桨毂速度，再用转换矩阵转到桨毂系
%     V_H = T_H2NAC' * T_NAC2B' * (V_body + Omega_skew * [x_BH; y_BH; z_BH]);
     V_H = T_H2NAC' * T_NAC2B' * (V_body );

    % ========== 计算前进比和旋翼侧滑角 ==========
    % 注意：如果处于纯悬停，V_H(1)和V_H(2)为0，计算beta_w时需防止分母为0
    V_xy = sqrt(V_H(1)^2 + V_H(2)^2);
    mu = V_xy / Omega_R;
    
    if V_xy < 1e-5
        beta_w = 0; % 悬停时无明显侧滑角
    else
        beta_w = asin(V_H(2) / V_xy);
    end

    % ========== 调用独立的迭代函数求解入流比和诱导速度 ==========
    V_z = V_H(3);
    [lamda, v_i] = calc_rotor_inflow(mu, V_z, Omega_R, CT);

end

== matlab function TRUAV_Dynamics_from_GTRS_trim/Force and Moments/body/Wing/MATLAB Function ==
  data: M_N input; B_c output; AR_w output; C_beta output; para input
function [B_c, AR_w, C_beta] = cWPara(M_N, para)
% computeWingParams 计算机翼气动压缩性因子、展弦比及C_beta系数
% 输入：
%   M_N         - 马赫数（无量纲）
%   Lambda_w_deg- 机翼后掠角（度）
%   b_w         - 翼展（m 或任意一致单位）
%   S_w         - 机翼面积（m^2 或任意一致单位）
% 输出：
%   B_c         - 压缩性因子，B_c = sqrt(1 - M_N^2 * cos^2(Lambda_w))
%   AR_w        - 展弦比，AR_w = b_w^2 / S_w
%   C_beta      - 侧滑相关系数，C_beta = (AR_w + 4*cos(Lambda_w)) / (AR_w*B_c + 4*cos(Lambda_w))
lambda_w =para(1);
b_w=para(2); S_w=para(3);

    % 将后掠角从度转换为弧度
       cos_L = cos(lambda_w);
    
    % 计算 B_c（注意避免根号内为负）
    inside = 1 - M_N^2 * cos_L^2;
    inside = abs(inside);
%     if inside < 0
%         error('马赫数和后掠角导致根号内为负，请检查输入：M_N * cos(Lambda_w) > 1');
%     end
    B_c = sqrt(inside);
    
    % 展弦比
    AR_w = b_w^2 / S_w;
    
    % C_beta 系数
    numerator = AR_w + 4 * cos_L;
    denominator = AR_w * B_c + 4 * cos_L;
%     if denominator == 0
%         error('分母为零，无法计算 C_beta');
%     end
    C_beta = numerator / denominator;
end

== matlab function TRUAV_Dynamics_from_GTRS_trim/Force and Moments/body/Wing/MATLAB Function2 ==
  data: common_vec output; V_flight output; para input; CG input; AC_w input; V_body input; pqr input; v_i_RL input; mu_RL input; tilt input; K_coeffs input; delta_F input; free_R output; delta_a input; free_L output; slip_R output; slip_L output
function [common_vec, V_flight, free_R, free_L, slip_R, slip_L] = w_pre(para, CG, AC_w, V_body, pqr, v_i_RL, mu_RL, tilt, K_coeffs, delta_F, delta_a)
    % 预处理模块：计算机翼气动状态参数（输出为列向量，无结构体）
    % ========== 参数提取 ==========
    rho = para(1); V_max = para(2); S_ws_max = para(3); S_wing_half = para(4)/2;
    i_w = para(5); c_w = para(6);
    K_FWO  = para(7); K_FWDF = para(8);
    b_w = para(9); a_sound = para(10);
    
    % 襟翼卸载增益
    delta_F_deg = abs(delta_F * (180/pi));
    K_FW = max(K_FWO - K_FWDF * delta_F_deg, 0.1);
    
    % 滑流区面积 (S_ws) 和自由流区面积 (S_free)
    V_flight = norm(V_body);
    vel_factor = max(0, (V_max - V_flight) / V_max);
    angle_term = sin(1.386 * (pi/2-tilt)) + cos(3.114 * (pi/2-tilt)); % tilt deg
    S_ws = S_ws_max * angle_term * vel_factor;
    S_ws = min(max(S_ws, 0), S_wing_half);

    if tilt >  pi/6
     S_ws = 0;
    end
    S_free = S_wing_half - S_ws;
    
    % 提取迎角修正系数
    K0 = K_coeffs(1); K1 = K_coeffs(2);
    
    % 旋翼诱导动压
    q_IWL = 0.5 * rho * v_i_RL(1)^2;
    q_IWR = 0.5 * rho * v_i_RL(2)^2;
    q_I_avg = (q_IWL + q_IWR) / 2;
    
    % 【修改 1】：公共参数向量改为列向量 (10x1) -> 使用分号 ;
    common_vec = [rho; S_wing_half; S_free; S_ws; K_FW; b_w; c_w; q_I_avg; delta_a; delta_F];
    
    % 左右翼气动中心
    AC_R = AC_w;
    AC_L = [AC_w(1); -AC_w(2); AC_w(3)];
    wings = {AC_R, AC_L};
    
    % 【修改 2】：初始化输出向量改为列向量 (N x 1)
    free_R = zeros(12, 1);
    free_L = zeros(12, 1);
    slip_R = zeros(4, 1);
    slip_L = zeros(4, 1);
    
    for i = 1:2
        AC = wings{i};
        r_ac_x = CG(1) - AC(1); % FS重心 - FS气动中心 (机翼在前，X为正)
        r_ac_y = AC(2) - CG(2); % BL气动中心 - BL重心 (右翼在右，Y为正)
        r_ac_z = CG(3) - AC(3); % WL重心 - WL气动中心 (机翼在上，Z为负)
        
        r_ac = [r_ac_x; r_ac_y; r_ac_z];
        
        % 自由流区速度
        V_local_free = V_body + cross(pqr, r_ac);
        u_f = V_local_free(1); v_f = V_local_free(2); w_f = V_local_free(3);
        V_mag_f = norm(V_local_free);
        
        if V_mag_f < 0.1
            alpha_f = 0; beta_f = 0; q_wfs = 0; Mach = 0;
        else
            alpha_f = atan2(w_f, u_f);
            beta_f  = asin(max(min(v_f/V_mag_f,1),-1));
            q_wfs   = 0.5 * rho * (u_f^2 + w_f^2);
            Mach    = V_mag_f / a_sound;
        end
        
        alpha_WFS = alpha_f + i_w;
        
        % 阻尼系数
        if V_mag_f > 0.1
            damping = b_w / (2 * V_mag_f);
        else
            damping = 0;
        end
        
        % 风轴角速率
        p_W = pqr(1)*cos(alpha_f)*cos(beta_f) + pqr(2)*sin(beta_f) + pqr(3)*sin(alpha_f)*cos(beta_f);
        r_W = -pqr(1)*sin(alpha_f) + pqr(3)*cos(alpha_f);
        
        % 【修改 3】：组装自由流状态向量改为列向量 (12x1) -> 使用分号 ;
        free_state = [alpha_WFS; beta_f; Mach; q_wfs; damping; p_W; r_W; alpha_f; beta_f; r_ac(1); r_ac(2); r_ac(3)];
        
        % 滑流区状态
        v_i_current = v_i_RL(i);
        mu_current = mu_RL(i);
        v_iW = (K0 + K1*mu_current) * v_i_current;
        V_wake_body = [v_iW * sin(tilt); 0; -v_iW * cos(tilt)];
        V_local_slip = V_local_free + V_wake_body;
        
        u_s = V_local_slip(1); v_s = V_local_slip(2); w_s = V_local_slip(3);
        V_mag_s = norm(V_local_slip);
        
        if V_mag_s < 0.1
            alpha_s = 0; beta_s = 0; q_s = 0; Mach_slip = 0;
        else
            alpha_s = atan2(w_s, u_s) + i_w;
            beta_s  = asin(max(min(v_s/V_mag_s,1),-1));
            q_s     = 0.5 * rho * V_mag_s^2;
            Mach_slip    = V_mag_f / a_sound;
        end
        
        % 【修改 4】：组装滑流状态向量改为列向量 (4x1) -> 使用分号 ;
        slip_state = [alpha_s; beta_s; q_s;Mach_slip];
        
        % 存入对应输出
        if i == 1
            free_R = free_state;
            slip_R = slip_state;
        else
            free_L = free_state;
            slip_L = slip_state;
        end
    end
end

== matlab function TRUAV_Dynamics_from_GTRS_trim/Force and Moments/body/Wing/MATLAB Function3 ==
  data: common_vec input; F_b output; free_R input; free_L input; slip_R input; slip_L input; coeff_R input; coeff_L input; coeff_slip_R input; coeff_slip_L input; M_b output; coeff input
function [F_b, M_b] = w_force(common_vec, free_R, free_L, slip_R, slip_L, coeff_R, coeff_L, coeff_slip_R, coeff_slip_L, coeff)
    % 后处理模块：根据查表系数计算气动力/力矩（无结构体，全部向量输入）
    % 输入：
    %   common_vec    - 10个公共参数 [rho, S_wing_half, S_free, S_ws, K_FW, b_w, c_w, q_I_avg, delta_a, delta_F]
    %   free_R, free_L- 自由流状态向量 (12个) [alpha_WFS, beta, Mach, q_wfs, damping, p_W, r_W, alpha_f, beta_f, r_ac_x, r_ac_y, r_ac_z]
    %   slip_R, slip_L- 滑流状态向量 (3个) [alpha_s, beta_s, q_s]
    %   coeff_R       - 右翼自由流系数 [CL_fs, CD_fs, CY_eta, Cl_beta, Cm0, Cn0] (6个)
    %   coeff_L       - 左翼自由流系数 (6个)
    %   coeff_slip_R  - 右翼滑流区系数 [CL_s, CD_s] (2个)
    %   coeff_slip_L  - 左翼滑流区系数 (2个)
    % 输出：
    %   F_b, M_b      - 体轴系总力和力矩 [3x1]

    % 解析公共参数
    rho          = common_vec(1);
    S_wing_half  = common_vec(2);
    S_free       = common_vec(3);
    S_ws         = common_vec(4);
    K_FW         = common_vec(5);
    b_w          = common_vec(6);
    c_w          = common_vec(7);
%     q_I_avg      = common_vec(8);
q_wfst=free_R(4);
    q_I_avg = (slip_R(3) + slip_L(3))/2;
    delta_a      = common_vec(9);
    delta_F      = common_vec(10);   % 用于计算 CL6a

    % 副翼升力损失系数 C_L6a (根据襟翼偏度估算)
    % 实际应根据 δ_F 查表获得，此处示例公式
    CL_delta_a = coeff(1);

    % 将左右翼状态存入 cell 便于循环
    free_states = {free_R, free_L};
    slip_states = {slip_R, slip_L};
    coeffs_free = {coeff_R, coeff_L};
    coeffs_slip = {coeff_slip_R, coeff_slip_L};

    Total_Force = zeros(3,1);
    Total_Moment = zeros(3,1);
 
    for i = 1:2
        fs = free_states{i};    % 12个元素
        ss = slip_states{i};    % 3个元素
        cf = coeffs_free{i};    % 6个元素
        cs = coeffs_slip{i};    % 2个元素

        % 解包自由流状态
        alpha_WFS = fs(1); beta     = fs(2); Mach   = fs(3);
        q_wfs     = fs(4); damping  = fs(5); p_W    = fs(6);
        r_W       = fs(7); alpha_f  = fs(8); beta_f = fs(9);
        r_ac = fs(10:12);
        r_ac = r_ac(:);   % 强制变为列向量
        % 解包滑流状态
        alpha_s = ss(1); beta_s = ss(2); q_s = ss(3);

        % 解包气动系数
        CL_fs = cf(1); CD_fs = cf(2); CY_beta = cf(3); Cl_beta = cf(4); Cm0 = cf(5); Cn_beta = cf(6);
        CL_s  = cs(1); CD_s  = cs(2);

        % 横航向动导数（此处假设为0，实际可从其他查表获得）
        Clp = coeff(2);Clr = coeff(3);Cnp = coeff(4); Cnr = coeff(5); C_l_delta_a = coeff(6);
        C_n_delta_a = coeff(7);

        CYp = 0; CYr = 0; 
        % 组合动态导数
        CY_total = CY_beta * beta_f + damping * (CYp * p_W + CYr * r_W);
        % 注意：副翼效率中的 q_I_avg/q_wfs 防除零
        q_ratio = q_I_avg / max(q_wfs, 1e-6);
        Cl_total = Cl_beta * beta_f + damping * (Clp * p_W + Clr * r_W) + q_ratio * C_l_delta_a * rad2deg(delta_a);  % Cl_da示例
        Cn_total = Cn_beta * beta_f + damping * (Cnp * p_W + Cnr * r_W) + q_ratio * C_n_delta_a * rad2deg(delta_a);  % Cn_da示例

        Cl_delta_t=C_l_delta_a * rad2deg(delta_a);
        Cons_cl= q_wfs * S_wing_half * b_w ;

        % 自由流区力/力矩（PDF公式）
        Lift_f   = q_wfs * S_free * CL_fs - q_wfs * S_wing_half * CL_delta_a * abs(rad2deg(delta_a));
        Drag_f   = q_wfs * S_free * CD_fs;
        Pitch_f  = q_wfs * S_wing_half * c_w * Cm0;
        Side_f   = q_wfs * S_wing_half * CY_total;
        Roll_f   = q_wfs * S_wing_half * b_w * Cl_total;
        Yaw_f    = q_wfs * S_wing_half * b_w * Cn_total;

        Roll_t   = q_wfs * S_wing_half * b_w *Cl_delta_t;

        % 风轴系到体轴系转换（自由流区）
        sa = sin(alpha_f); ca = cos(alpha_f);
        sb = sin(beta_f);  cb = cos(beta_f);
        F_body_f = [-Drag_f*ca*cb - Side_f*ca*sb + Lift_f*sa;
                    -Drag_f*sb      + Side_f*cb;
                    -Drag_f*sa*cb - Side_f*sa*sb - Lift_f*ca];
        M_body_f = [ Roll_f*ca - Yaw_f*sa;
                     Pitch_f;
                     Roll_f*sa + Yaw_f*ca ];
        M_body_f = M_body_f + cross(r_ac, F_body_f);

        % 滑流区力/力矩
        Lift_s = q_s * S_ws * CL_s * K_FW;
        Drag_s = q_s * S_ws * CD_s * K_FW;
        % 滑流区侧力假设为0
        sa_s = sin(alpha_s); ca_s = cos(alpha_s);
        sb_s = sin(beta_s);  cb_s = cos(beta_s);
        F_body_s = [-Drag_s*ca_s*cb_s + Lift_s*sa_s;
                    -Drag_s*sb_s;
                    -Drag_s*sa_s*cb_s - Lift_s*ca_s];
        M_body_s = cross(r_ac, F_body_s);

        % 累加
        Total_Force = Total_Force + F_body_f + F_body_s;
        Total_Moment = Total_Moment + M_body_f + M_body_s;
    end

    F_b = Total_Force;
    M_b = Total_Moment;
end

== matlab function TRUAV_Dynamics_from_GTRS_trim/Force and Moments/body/Wing/Mach ==
  data: para input; V_body input; Mach_N output
function Mach_N = vtail_prep(para, V_body)
    % =====================================================================
    % 垂尾拆分模块 1：状态预处理 (算出马赫数，用于驱动第一级 X_Kr 查表)
    % =====================================================================
    a_sound = para(4); % 提取音速
    Mach_N = norm(V_body) / a_sound;
end

== matlab function TRUAV_Dynamics_from_GTRS_trim/Force and Moments/Inertia moment and CG/MATLAB Function ==
  data: beta_m input; CG output; Pos input
function CG  = fcn(beta_m, Pos)

% ========== 固定常数（从报告表格中提取）==========
% 短舱参数（两个短舱总重）
W_P = 4200;        % 两个短舱总重 [lbs]

% 直升机模式下的初始重心（β_m = 0°）
SL_CG_0 = Pos(1);   % 初始纵向重心 [in]（前重心状态）
BL_CG = Pos(2);
WL_CG_0 = Pos(3);   % 初始垂向重心 [in]


% 短舱重心位置（Pylon CG）
SL_P = Pos(4);      % 短舱重心纵向位置 [in]
% BL_P = Pos(5);      % 短舱重心垂向位置 [in]
WL_P = Pos(6);      % 短舱重心垂向位置 [in]

% 旋翼轴枢轴点位置（Shaft Pivot Point）
SL_SP = Pos(7);     % 枢轴点纵向位置 [in]
% BL_SP = Pos(8);     % 枢轴点纵向位置 [in]
WL_SP = Pos(9);     % 枢轴点垂向位置 [in]
% L_n = Pos(10);  
%  倾转机总重量
GW =13000;

% ========== 计算重量比和偏移量 ==========
% 重量比
W_ratio = W_P / GW;

% 纵向偏移 X = (W_P/GW) * (SL_SP - SL_P) / 12
X = W_ratio * (SL_SP - SL_P) / 12;   % [ft]

% 垂向偏移 Z = (W_P/GW) * (WL_SP - WL_P) / 12
Z = W_ratio * (WL_SP - WL_P) / 12;   % [ft]

% ========== 角度转换 ==========
% 输入为度数，转换为弧度
beta_rad = beta_m ;

% ========== 计算重心变化量 ==========
% 纵向变化：X_CG = Z * sinβ + X * (1 - cosβ)
X_CG = Z * sin(beta_rad) + X * (1 - cos(beta_rad));   % [ft]

% 垂向变化：Z_CG = Z * (1 - cosβ) - X * sinβ
Z_CG = Z * (1 - cos(beta_rad)) - X * sin(beta_rad);    % [ft]

% ========== 计算最终重心位置 ==========
% 转换回英寸并加上初始值
SL_CG = SL_CG_0 + 12 * X_CG;   % [in]
WL_CG = WL_CG_0 + 12 * Z_CG;   % [in]

%===========输出====
CG=[SL_CG;BL_CG;WL_CG];

end

== matlab function TRUAV_Dynamics_from_GTRS_trim/Feedback/MATLAB Function1 ==
  data: vxyz input; course output; gndSpeed output
function [course, gndSpeed] = fcn(vxyz)

vx = vxyz(1);
vy = vxyz(2);
course = atan2(vy, vx);
gndSpeed = norm([vx vy 0]);
